simulink model "InputSimulationFromWorkSpace"  (R2016b)
settings: Solver=FixedStepDiscrete  StartTime=0.0  StopTime=inf  FixedStep=sCoreParams.core.stepPeriod  RelTol=1e-3  EnableMultiTasking=on
undefined symbols (not defined in the file): sCoreParams
libraries: simulink x1, dspsrcs4 x1
settings Model: Creator=rzelmann  LastModifiedBy=Rina
settings SolverCC: EnableConcurrentExecution=on  ConcurrentTasks=on  AutoInsertRateTranBlk=on  InsertRTBMode=Always
settings DataIOCC: SaveFormat=StructureWithTime  SaveOutput=off  SignalLogging=off  DSMLogging=off  SaveTime=off
settings OptimizationCC: BlockReduction=off  OptimizeBlockIOStorage=off  BufferReuse=off  GlobalBufferReuse=off  ExpressionFolding=off  LocalBlockOutputs=off
settings HardwareCC: ProdBitPerPointer=32  ProdBitPerSizeT=32  ProdBitPerPtrDiffT=32  ProdLargestAtomicFloat=None  ProdWordSize=32  ProdLongLongMode=on  ProdHWDeviceType=Generic->32-bit x86 compatible
settings RTWCC: SystemTargetFile=slrt.tlc  TemplateMakefile=slrt_default_tmf  Description=Simulink Real-Time  RTWCompilerOptimization=on

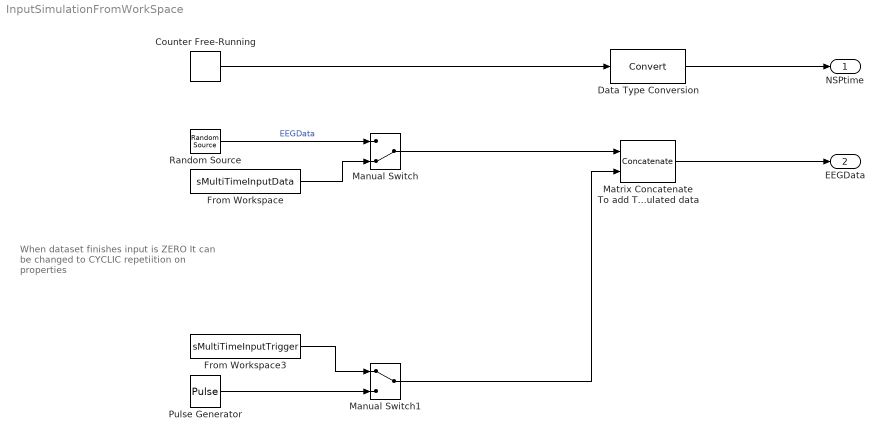
== system InputSimulationFromWorkSpace ==
  note: When dataset finishes input is ZERO
      | It can be changed to CYCLIC repetiition
      | on properties
  Counter Free-Running : simulink/Sources/Counter Free-Running  NumBits=64  tsamp=sCoreParams.core.stepPeriod
  Data Type Conversion : DataTypeConversion
  From Workspace : FromWorkspace  VariableName=sMultiTimeInputData  SampleTime=sCoreParams.core.stepPeriod  Interpolate=off  OutputAfterFinalValue=Setting to zero
  From Workspace3 : FromWorkspace  VariableName=sMultiTimeInputTrigger  SampleTime=sCoreParams.core.stepPeriod  Interpolate=off  OutputAfterFinalValue=Setting to zero
  Manual Switch : ManualSwitch  CurrentSetting=0
  Manual Switch1 : ManualSwitch
  Matrix Concatenate To add Trigger after simulated data : Concatenate  Mode=Multidimensional array  ConcatenateDimension=2
  Pulse Generator : DiscretePulseGenerator  Amplitude=ones(sCoreParams.core.samplesPerStep, 2)  Period=sCoreParams.core.samplingRate * 10  SampleTime=-1  VectorParams1D=off
  Random Source : dspsrcs4/Random Source  SrcType=Uniform  NormMethod=Ziggurat  CltLength=12  MinVal=-10 * ones(1, sCoreParams.core.maxChannelsAllNSPs-2)  MaxVal=10 * ones(1, sCoreParams.core.maxChannelsAllNSPs-2)  MeanVal=0  VarVal=1  RepMode=Not repeatable  rawSeed=1  IsInherit=off  SampMode=Discrete  SampTime=-1  SampFrame=sCoreParams.core.samplesPerStep  DataType=Double  OutComplex=Real  OutputFrames=off
  NSPtime : Outport
  EEGData : Outport  Port=2
  wires:
  Manual Switch/1 -> Matrix Concatenate To add Trigger after simulated data/1
  Counter Free-Running/1 -> Data Type Conversion/1
  Data Type Conversion/1 -> NSPtime/1
  Matrix Concatenate To add Trigger after simulated data/1 -> EEGData/1
  From Workspace/1 -> Manual Switch/2
  From Workspace3/1 -> Manual Switch1/1
  Manual Switch1/1 -> Matrix Concatenate To add Trigger after simulated data/2
  Random Source/1 -> Manual Switch/1  "EEGData"
  Pulse Generator/1 -> Manual Switch1/2
